simulink model "ex1_controller_fulltank"  (R2020a)
settings: Solver=VariableStepAuto  StartTime=0.0  StopTime=100  RelTol=1e-3
settings Model: Creator=mumun  LastModifiedBy=mumun

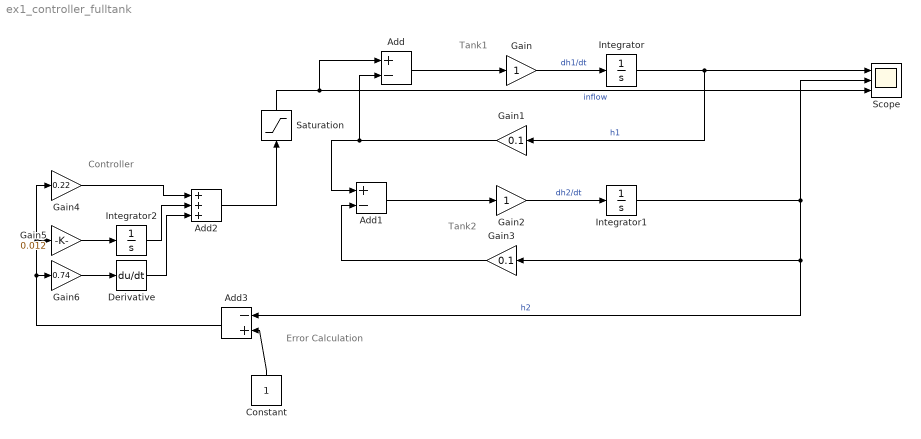
== system ex1_controller_fulltank ==
  note: Error Calculation
  note: Tank2
  note: Tank1
  note: Controller
  Add : Sum  Inputs=+-
  Add1 : Sum  Inputs=+-
  Add2 : Sum  Inputs=+++
  Add3 : Sum  Inputs=-+
  Constant : Constant
  Derivative : Derivative
  Gain : Gain
  Gain1 : Gain  Gain=0.1
  Gain2 : Gain
  Gain3 : Gain  Gain=0.1
  Gain4 : Gain  Gain=0.22
  Gain5 : Gain  Gain=0.012
  Gain6 : Gain  Gain=0.74
  Integrator : Integrator  InitialCondition=2  UpperSaturationLimit=2  LowerSaturationLimit=0
  Integrator1 : Integrator  InitialCondition=2  UpperSaturationLimit=2  LowerSaturationLimit=0
  Integrator2 : Integrator  LowerSaturationLimit=0
  Saturation : Saturate  UpperLimit=inf  LowerLimit=0
  Scope : Scope  NumInputPorts=3
  wires:
  Add/1 -> Gain/1
  Gain/1 -> Integrator/1  "dh1/dt"
  Gain1/1 -> Add1/1, Add/2
  Integrator/1 -> Gain1/1, Scope/1  "h1"
  Add1/1 -> Gain2/1
  Gain2/1 -> Integrator1/1  "dh2/dt"
  Gain3/1 -> Add1/2
  Integrator1/1 -> Add3/1, Gain3/1, Scope/2  "h2"
  Constant/1 -> Add3/2
  Gain5/1 -> Integrator2/1
  Gain4/1 -> Add2/1
  Integrator2/1 -> Add2/2
  Add2/1 -> Saturation/1
  Gain6/1 -> Derivative/1
  Derivative/1 -> Add2/3
  Add3/1 -> Gain6/1, Gain5/1, Gain4/1
  Saturation/1 -> Add/1, Scope/3  "inflow"
